simulink model "Aircraft6dof_forTrimAndLin_ATT_wInputs"  (R2025b)
settings: Solver=ode4  StartTime=startTime  StopTime=stopTime  FixedStep=stepTime  RelTol=1e-3  EnableMultiTasking=on
values from neighbouring files (symbols this model uses):
  InitAtt = InitAtt_deg * deg2rad    [Setup_A8_master.m]
  InitPos = A8.init.InitPos    [Setup_A8_master.m]
  om_motor_init = 0    [Setup_A8_master.m]
  omDot_motor = 0    [Setup_A8_master.m]
undefined symbols (not defined in the file or in its folder): a0_s2, a0_s3, a0_s4, a0_s5, AR_s2, AR_s3, AR_s4, AR_s5, c_s2, c_s3, c_s4, c_s5, CD0_s2, CD0_s3, CD0_s4, CD0_s5, CDa_s2, CDa_s3, CDa_s4, CDa_s5, CL0_s2, CL0_s3, CL0_s4, CL0_s5, CM0_s2, CM0_s3, CM0_s4, CM0_s5, CMa_s2, CMa_s3, CMa_s4, CMa_s5, dCL_du, dE_0, dEL_0, dER_0, dR_0, e_s2, e_s3, e_s4, e_s5, g_E_N, i_s2, i_s3, i_s4, i_s5, InitQuat, InitRates, InitVel, J, J_int, m, MixMatrix, n_int, n_s2, n_s3, n_s4, n_s5, S_s2, S_s3 ... (+16)
libraries: vrlib x7, simulink x3
(part 2 of 2)

== system Aircraft6dof_forTrimAndLin_ATT_wInputs/Equations Of Motion State Equations/Rot Kin (Orientation) Euler/Integrate ==
  AttDot : Inport
  Constant1 : Constant  Value=InitAtt
  Demux : Demux  Outputs=3
  Demux1 : Demux  Outputs=3
  Mux : Mux  Inputs=3
  Phi : Integrator  InitialConditionSource=external
  Psi : Integrator  InitialConditionSource=external
  Theta : Integrator  InitialConditionSource=external
  Att : Outport  PortDimensions=3
  wires:
  Demux1/1 -> Phi/2
  Phi/1 -> Mux/1
  Demux/3 -> Psi/1
  Demux1/3 -> Psi/2
  Demux1/2 -> Theta/2
  Theta/1 -> Mux/2
  Demux/2 -> Theta/1
  Mux/1 -> Att/1
  Constant1/1 -> Demux1/1
  AttDot/1 -> Demux/1
  Demux/1 -> Phi/1
  Psi/1 -> Mux/3

== system Aircraft6dof_forTrimAndLin_ATT_wInputs/Equations Of Motion State Equations/Rot Kin (Orientation) Quaternion/QuatMult ==
  q : Inport
  r : Inport  Port=2
  Mux1 : Mux
  q0 : Subsystem
  q1 : Subsystem
  q2 : Subsystem
  q4 : Subsystem
  q*r : Outport
  wires:
  q/1 -> q4/1(q), q2/1(q), q1/1(q), q0/1(q)
  Mux1/1 -> q*r/1
  q0/1(q0) -> Mux1/1
  q4/1(q3) -> Mux1/4
  q1/1(q1) -> Mux1/2
  q2/1(q2) -> Mux1/3
  r/1 -> q4/2(r), q2/2(r), q1/2(r), q0/2(r)

== system Aircraft6dof_forTrimAndLin_ATT_wInputs/Equations Of Motion State Equations/Rot Kin (Orientation) Quaternion/norm1 ==
  q : Inport
  Dot Product : DotProduct  OutDataTypeStr=Inherit: Inherit via internal rule
  Math Function : Math  Operator=sqrt  SignedPower=on
  e/|e| : Product  Inputs=*/  InputSameDT=on  RndMeth=Zero  SaturateOnIntegerOverflow=on  OutDataTypeStr=Inherit: Same as first input
  q/|q| : Outport
  wires:
  e/|e|/1 -> q/|q|/1
  Math Function/1 -> e/|e|/2
  Dot Product/1 -> Math Function/1
  q/1 -> e/|e|/1, Dot Product/1, Dot Product/2

== system Aircraft6dof_forTrimAndLin_ATT_wInputs/Equations Of Motion State Equations/Trans Dyn (Forces)/Integrate ==
  VelDot : Inport
  Constant2 : Constant  Value=InitVel
  Demux : Demux  Outputs=3
  Demux1 : Demux  Outputs=3
  Mux : Mux  Inputs=3
  U : Integrator  InitialConditionSource=external
  V : Integrator  InitialConditionSource=external
  W : Integrator  InitialConditionSource=external
  Vel : Outport
  wires:
  Demux1/1 -> U/2
  U/1 -> Mux/1
  Demux/3 -> W/1
  Demux1/3 -> W/2
  Demux1/2 -> V/2
  V/1 -> Mux/2
  Demux/2 -> V/1
  Mux/1 -> Vel/1
  Constant2/1 -> Demux1/1
  VelDot/1 -> Demux/1
  Demux/1 -> U/1
  W/1 -> Mux/3

== system Aircraft6dof_forTrimAndLin_ATT_wInputs/Equations Of Motion State Equations/Trans Kin (Spherical)/LatDot ==
  Vn : Inport
  Rearth : Inport  Port=2
  alt : Inport  Port=3
  Add : Sum
  Divide : Product  Inputs=*/
  latDot : Outport
  wires:
  Vn/1 -> Divide/1
  Add/1 -> Divide/2
  Divide/1 -> latDot/1
  alt/1 -> Add/2
  Rearth/1 -> Add/1

== system Aircraft6dof_forTrimAndLin_ATT_wInputs/Equations Of Motion State Equations/Trans Kin (Spherical)/LonDot ==
  Ve : Inport
  Rearth : Inport  Port=2
  alt : Inport  Port=3
  lat : Inport  Port=4
  Add1 : Sum
  Divide1 : Product  Inputs=*//
  Trigonometric Function : Trigonometry  Operator=cos
  lonDot : Outport
  wires:
  Ve/1 -> Divide1/1
  Add1/1 -> Divide1/2
  lat/1 -> Trigonometric Function/1
  Trigonometric Function/1 -> Divide1/3
  Divide1/1 -> lonDot/1
  Rearth/1 -> Add1/1
  alt/1 -> Add1/2

== system Aircraft6dof_forTrimAndLin_ATT_wInputs/Equations Of Motion State Equations/Trans Kin (Spherical)/wrap lon ==
  lon : Inport
  Add : Sum  Inputs=-+
  Add1 : Sum
  Compare To Constant : simulink/Logic and Bit Operations/Compare To Constant  relop=>  const=pi  OutDataTypeStr=boolean
  Compare To Constant1 : simulink/Logic and Bit Operations/Compare To Constant  relop=<=  const=-pi  OutDataTypeStr=boolean
  Constant : Constant  Value=2*pi
  Switch : Switch  Criteria=u2 > Threshold  SaturateOnIntegerOverflow=off  InputSameDT=off
  Switch1 : Switch  Criteria=u2 > Threshold  SaturateOnIntegerOverflow=off  InputSameDT=off
  -pi < lon <= pi : Outport
  wires:
  lon/1 -> Compare To Constant/1, Add/2, Switch/3
  Add/1 -> Switch/1
  Compare To Constant/1 -> Switch/2
  Compare To Constant1/1 -> Switch1/2
  Switch/1 -> Switch1/3, Add1/2, Compare To Constant1/1
  Switch1/1 -> -pi < lon <= pi/1
  Constant/1 -> Add/1, Add1/1
  Add1/1 -> Switch1/1

== system Aircraft6dof_forTrimAndLin_ATT_wInputs/Equations Of Motion State Equations/Rot Dyn (Moments)/Internal Rotational Component 01/Integrate ==
  hInt_dot : Inport
  J : Inport  Port=2
  n : Inport  Port=3
  Constant2 : Constant  Value=om_motor_init
  Demux : Demux  Outputs=3
  Demux1 : Demux  Outputs=3
  Mux : Mux  Inputs=3
  Product1 : Product  Inputs=3
  hx : Integrator  InitialConditionSource=external
  hy : Integrator  InitialConditionSource=external
  hz : Integrator  InitialConditionSource=external
  hInt : Outport
  wires:
  Demux1/1 -> hx/2
  hx/1 -> Mux/1
  Demux/3 -> hz/1
  Demux1/3 -> hz/2
  Demux1/2 -> hy/2
  hy/1 -> Mux/2
  Demux/2 -> hy/1
  Mux/1 -> hInt/1
  Product1/1 -> Demux1/1
  hInt_dot/1 -> Demux/1
  Demux/1 -> hx/1
  hz/1 -> Mux/3
  Constant2/1 -> Product1/3
  n/1 -> Product1/2
  J/1 -> Product1/1

== system Aircraft6dof_forTrimAndLin_ATT_wInputs/Equations Of Motion State Equations/Rot Kin (Orientation) Quaternion/QuatMult/q0 ==
  q : Inport
  r : Inport  Port=2
  Demux : Demux
  Demux1 : Demux
  Product{,1..3} (4 alike) : Product  RndMeth=Zero
  Sum : Sum  Inputs=+---
  q0 : Outport
  wires:
  Product2/1 -> Sum/3
  Sum/1 -> q0/1
  Product3/1 -> Sum/4
  Product1/1 -> Sum/2
  Product/1 -> Sum/1
  Demux/4 -> Product3/1
  Demux1/4 -> Product3/2
  Demux1/3 -> Product2/2
  Demux/3 -> Product2/1
  Demux1/2 -> Product1/2
  Demux/2 -> Product1/1
  Demux1/1 -> Product/2
  Demux/1 -> Product/1
  r/1 -> Demux1/1
  q/1 -> Demux/1

== system Aircraft6dof_forTrimAndLin_ATT_wInputs/Equations Of Motion State Equations/Rot Kin (Orientation) Quaternion/QuatMult/q1 ==
  q : Inport
  r : Inport  Port=2
  Demux : Demux
  Demux1 : Demux
  Product{,1..3} (4 alike) : Product  RndMeth=Zero
  Sum : Sum  Inputs=+++-
  q1 : Outport
  wires:
  Demux1/3 -> Product3/2
  Demux1/4 -> Product2/2
  Demux1/1 -> Product1/2
  Demux1/2 -> Product/2
  q/1 -> Demux/1
  r/1 -> Demux1/1
  Demux/1 -> Product/1
  Demux/2 -> Product1/1
  Demux/3 -> Product2/1
  Demux/4 -> Product3/1
  Product/1 -> Sum/1
  Product1/1 -> Sum/2
  Product3/1 -> Sum/4
  Sum/1 -> q1/1
  Product2/1 -> Sum/3

== system Aircraft6dof_forTrimAndLin_ATT_wInputs/Equations Of Motion State Equations/Rot Kin (Orientation) Quaternion/QuatMult/q2 ==
  q : Inport
  r : Inport  Port=2
  Demux : Demux
  Demux1 : Demux
  Product{,1..3} (4 alike) : Product  RndMeth=Zero
  Sum : Sum  Inputs=+-++
  q2 : Outport
  wires:
  Demux1/2 -> Product3/2
  Demux1/1 -> Product2/2
  Demux1/4 -> Product1/2
  Demux1/3 -> Product/2
  Product2/1 -> Sum/3
  Sum/1 -> q2/1
  Product3/1 -> Sum/4
  Product1/1 -> Sum/2
  Product/1 -> Sum/1
  Demux/4 -> Product3/1
  Demux/3 -> Product2/1
  Demux/2 -> Product1/1
  r/1 -> Demux1/1
  q/1 -> Demux/1
  Demux/1 -> Product/1

== system Aircraft6dof_forTrimAndLin_ATT_wInputs/Equations Of Motion State Equations/Rot Kin (Orientation) Quaternion/QuatMult/q4 ==
  q : Inport
  r : Inport  Port=2
  Demux : Demux
  Demux1 : Demux
  Product{,1..3} (4 alike) : Product  RndMeth=Zero
  Sum : Sum  Inputs=++-+
  q3 : Outport
  wires:
  Demux1/4 -> Product/2
  Demux1/3 -> Product1/2
  Demux1/1 -> Product3/2
  Demux1/2 -> Product2/2
  q/1 -> Demux/1
  r/1 -> Demux1/1
  Demux/1 -> Product/1
  Demux/2 -> Product1/1
  Demux/3 -> Product2/1
  Demux/4 -> Product3/1
  Product/1 -> Sum/1
  Product1/1 -> Sum/2
  Product3/1 -> Sum/4
  Sum/1 -> q3/1
  Product2/1 -> Sum/3

== matlab function Aircraft6dof_forTrimAndLin_ATT_wInputs/Atmosphere Model/Standard Atmosphere - Troposphere ==
  data: h input; rho output
function rho = fcn(h)
%#codegen

temp_C = 15.04 - 0.00649 * h;
temp_K = 273.15 + temp_C;

press_NQm2 = 101.29 * (temp_K/288.08)^5.256;

rho_kgQm3 = press_NQm2 / (0.2869 *temp_K);

rho = rho_kgQm3;

== matlab function Aircraft6dof_forTrimAndLin_ATT_wInputs/Equations Of Motion State Equations/Rot Dyn (Moments)/inv of matrix ==
  data: u input; y output
function y = fcn(u)
%#codegen

y = inv(u);

== matlab function Aircraft6dof_forTrimAndLin_ATT_wInputs/Compute Wind Axes Vector/Compute Wind DCMs ==
  data: Vinf input; C_SB output; C_WB output; alpha input; beta input
function [C_SB, C_WB] = fcn(Vinf, alpha, beta)
%#codegen

C_SB = [cos(alpha)   0   sin(alpha) ;
        0           1   0         ;
        -sin(alpha)  0   cos(alpha)];
    
C_WS = [cos(beta)   sin(beta)   0 ;
        -sin(beta)  cos(beta)   0 ;
        0           0           1];
C_WB = C_WS * C_SB;

== matlab function Aircraft6dof_forTrimAndLin_ATT_wInputs/Equations Of Motion State Equations/Rot Kin (Orientation) Euler/MATLAB Function ==
  data: ATT input; MATRIX output
function MATRIX = EulerIntegrationMatrix(ATT)
%#codegen

phi=ATT(1);
theta=ATT(2);
psi=ATT(3);

MATRIX = [1     sin(phi)*tan(theta)   cos(phi)*tan(theta) ; 
          0     cos(phi)             -sin(phi)            ;
          0     sin(phi)/cos(theta)   cos(phi)/cos(theta)   ];

== matlab function Aircraft6dof_forTrimAndLin_ATT_wInputs/Equations Of Motion State Equations/MATLAB Function ==
  data: ATT input; DCM output
function DCM = ATT2DCM(ATT)
%#codegen

phi=ATT(1);
theta=ATT(2);
psi=ATT(3);

DCM = [ cos(theta)*cos(psi)                             cos(theta)*sin(psi)                            -sin(theta)          ; 
        sin(theta)*cos(psi)*sin(phi)-sin(psi)*cos(phi)  sin(theta)*sin(psi)*sin(phi)+cos(psi)*cos(phi)  cos(theta)*sin(phi) ;
        sin(theta)*cos(psi)*cos(phi)+sin(psi)*sin(phi)  sin(theta)*sin(psi)*cos(phi)-cos(psi)*sin(phi)  cos(theta)*cos(phi)   ];
